simulink model "untitled"  (R2018a)
settings: Solver=FixedStepAuto  StartTime=0.0  StopTime=5  FixedStep=0.001  RelTol=1e-3
settings Model: Creator=ahmed  LastModifiedBy=ahmed

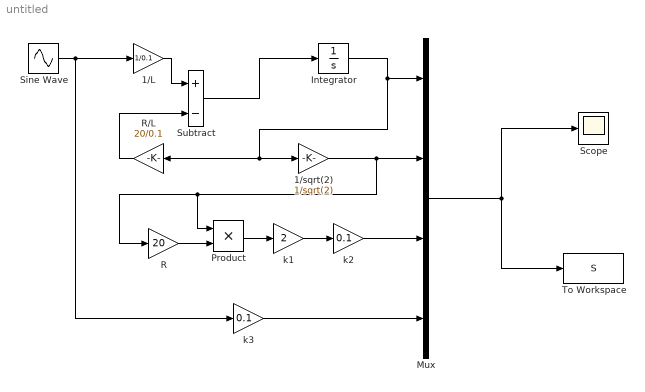
== system untitled ==
  1/L : Gain  Gain=1/0.1
  1/sqrt(2) : Gain  Gain=1/sqrt(2)
  Integrator : Integrator
  Mux : Mux
  Product : Product
  R : Gain  Gain=20
  R/L : Gain  Gain=20/0.1
  Scope : Scope
  Sine Wave : Sin  SampleTime=0
  Subtract : Sum  Inputs=+-
  To Workspace : ToWorkspace  VariableName=S  SaveFormat=Structure  SampleTime=-1
  k1 : Gain  Gain=2
  k2 : Gain  Gain=0.1
  k3 : Gain  Gain=0.1
  wires:
  Mux/1 -> To Workspace/1, Scope/1
  Sine Wave/1 -> k3/1, 1/L/1
  1/L/1 -> Subtract/1
  Integrator/1 -> 1/sqrt(2)/1, R/L/1, Mux/1
  R/L/1 -> Subtract/2
  Subtract/1 -> Integrator/1
  1/sqrt(2)/1 -> Product/1, R/1, Mux/2
  k3/1 -> Mux/4
  R/1 -> Product/2
  k1/1 -> k2/1
  Product/1 -> k1/1
  k2/1 -> Mux/3
